simulink model "Demo"  (Simulink 6.2)
settings: Solver=ode45  StartTime=0.0  StopTime=10.0  RelTol=1e-3
settings Model: LastModifiedBy=suarezjl
settings DataIOCC: SignalLoggingName=sigsOut
settings HardwareCC: TargetUnknown=on

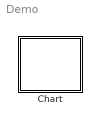
== system Demo ==
  Chart : Stateflow chart

== stateflow chart Chart ==
  state StartCameras
    \\Sally\HeadTrackingDemo\HeadModule\HeadAgent\EyeMotionControl.Initialize()
    \\Sally\HeadTrackingDemo\DemoStateMachine.Wait(1000)
    \\Sally\HeadTrackingDemo\HeadModule\LeftCameraAgent\StateMachine.LoadSM()
    \\Sally\HeadTrackingDemo\HeadModule\LeftCameraAgent\StateMachine.Start()
    \\Sally\HeadTrackingDemo\HeadModule\RightCameraAgent\StateMachine.LoadSM()
    \\Sally\HeadTrackingDemo\HeadModule\RightCameraAgent\StateMachine.Start()
    \\Sally\HeadTrackingDemo\DemoStateMachine.Wait(2500)
  state StartHead
    \\Sally\HeadTrackingDemo\HeadModule\HeadAgent\StateMachine.LoadSM()
    \\Sally\HeadTrackingDemo\HeadModule\HeadAgent\StateMachine.Start()
  state Stop
    \\Sally\HeadTrackingDemo\HeadModule\HeadAgent\StateMachine.Stop()
    \\Sally\HeadTrackingDemo\HeadModule\LeftCameraAgent\StateMachine.Stop()
    \\Sally\HeadTrackingDemo\HeadModule\RightCameraAgent\StateMachine.Stop()
  (default) -> StartCameras : Start
  StartCameras -> StartHead : Always
  StartHead -> Stop : Signal="Stop"
